simulink model "DI"  (R2015b)
settings: Solver=VariableStepAuto  StartTime=0.0  StopTime=10.0  RelTol=1e-3
settings Model: Creator=Pramod  LastModifiedBy=Pramod

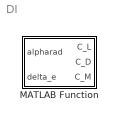
== system DI ==
  MATLAB Function : MATLAB Function  TreatAsAtomicUnit=on

== matlab function DI/MATLAB Function ==
  data: alpharad input; C_L output; delta_e input; C_D output; C_M output
function [C_L,C_D,C_M] = fcn(alpharad, delta_e)
g = 9.8;
rho = 1.225;
%q=0
%y(4)=0 % for level flight
m = 1043.26;
C_bar = 1.493;
b = 10.911;
S_ref = 16.1651;
C_L_0 = 0.25;
C_L_alpha = 4.47;
C_L_q = 1.7;
C_L_delta_e = 0.3476;
C_M_0 = -0.02;
C_M_alpha = -1.8;
C_M_alpha_dot = -12.4;
C_M_delta_e = -1.28;
C_L = C_L_0 + C_L_alpha*alpharad +   C_L_delta_e*delta_e;
C_D = C_D_0 + k*C_L^2;
C_M = C_M_0 + C_M_alpha*alpharad +  C_M_delta_e*delta_e;
C_X = -C_D*cos(alpharad) + C_L*sin(alpharad);
C_Z = -C_D*sin(alpharad) - C_L*cos(alpharad);

y = u;
